simulink model "try1"  (R2013a)
settings: Solver=ode45  StartTime=0.0  StopTime=10.0  RelTol=1e-3
values from neighbouring files (symbols this model uses):
  g = 9.82    [Untitled.m]
  kt = (stall_torque*rm)/max_volt    (= 0.302166666667)    [Untitled.m]
  kv = (stall_torque*rm)/(kt*max_omega)    (= 0.572957795131)    [Untitled.m]
  mp = mtot    (= 2.15528)    [Untitled.m]
  plant = c2d(plant,Ts)    [Untitled.m]
  rm = 7.4    [Untitled.m]
  rp = masscenter    (= 0.156968004157)    [Untitled.m]
undefined symbols (not defined in the file or in its folder): iw, k, kalmanL, kn
libraries: simulink x2
settings Model: Creator=user  LastModifiedBy=user

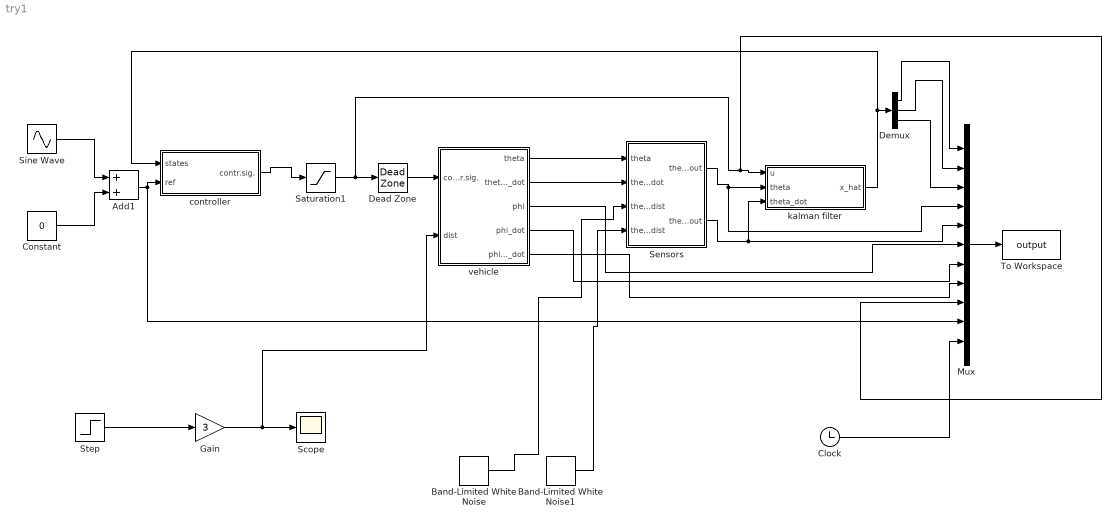
== system try1 ==
  Add1 : Sum
  Band-Limited White Noise : simulink/Sources/Band-Limited White Noise  Cov=[0.1]  Ts=0.1  seed=[23341]
  Band-Limited White Noise1 : simulink/Sources/Band-Limited White Noise  Cov=[0.1]  Ts=0.1  seed=[23341]
  Clock : Clock
  Constant : Constant  Value=0
  Dead Zone : DeadZone  SaturateOnIntegerOverflow=on
  Demux : Demux  Outputs=3
  Gain : Gain  Gain=3
  Mux : Mux  Inputs=11
  Saturation1 : Saturate
  Scope : Scope
  Sensors : Subsystem
  Sine Wave : Sin  SampleTime=0
  Step : Step  SampleTime=0
  To Workspace : ToWorkspace  VariableName=output  SampleTime=-1  SaveFormat=Timeseries
  controller : Subsystem
  kalman filter : Subsystem
  vehicle : Subsystem
  wires:
  Constant/1 -> Add1/2
  Sine Wave/1 -> Add1/1
  Add1/1 -> Mux/10, controller/2(ref)
  vehicle/1(theta) -> Sensors/1(theta)
  vehicle/2(theta_dot) -> Sensors/2(theta_dot)
  Band-Limited White Noise/1 -> Sensors/3(theta_dist)
  Band-Limited White Noise1/1 -> Sensors/4(theta_dot_dist)
  Demux/1 -> Mux/1
  Demux/2 -> Mux/2
  Demux/3 -> Mux/3
  Sensors/1(theta_out) -> Mux/4, kalman filter/2(theta)
  Sensors/2(theta_dot_out) -> kalman filter/3(theta_dot), Mux/5
  controller/1(contr.sig.) -> Saturation1/1
  Mux/1 -> To Workspace/1
  Clock/1 -> Mux/11
  Step/1 -> Gain/1
  Gain/1 -> vehicle/2(dist), Scope/1
  Dead Zone/1 -> vehicle/1(contr.sig.)
  vehicle/3(phi) -> Mux/6
  vehicle/4(phi_dot) -> Mux/7
  vehicle/5(phi_dot_dot) -> Mux/8
  kalman filter/1(x_hat) -> controller/1(states), Demux/1
  Saturation1/1 -> Dead Zone/1, Mux/9, kalman filter/1(u)

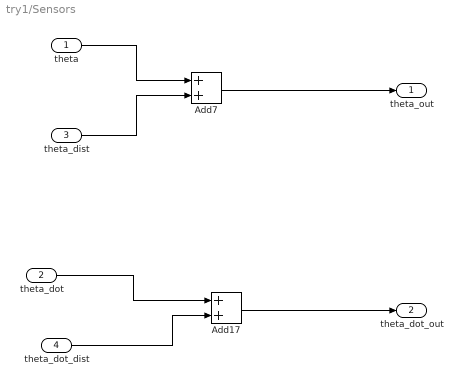
== system try1/Sensors ==
  theta : Inport
  theta_dot : Inport  Port=2
  theta_dist : Inport  Port=3
  theta_dot_dist : Inport  Port=4
  Add17 : Sum
  Add7 : Sum
  theta_out : Outport
  theta_dot_out : Outport  Port=2
  wires:
  theta/1 -> Add7/1
  theta_dist/1 -> Add7/2
  theta_dot/1 -> Add17/1
  theta_dot_dist/1 -> Add17/2
  Add7/1 -> theta_out/1
  Add17/1 -> theta_dot_out/1

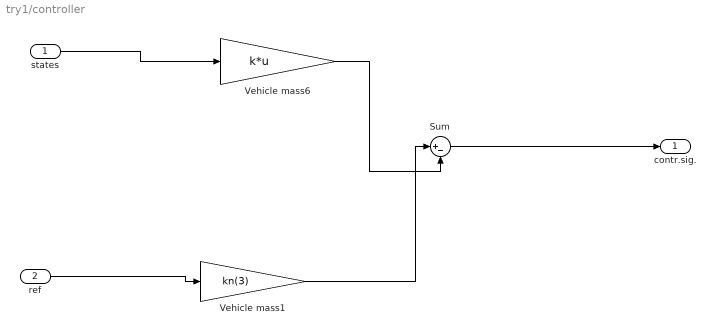
== system try1/controller ==
  states : Inport
  ref : Inport  Port=2
  Sum : Sum  Inputs=|+-
  "Vehicle mass1 " : Gain  Gain=kn(3)
  Vehicle mass6 : Gain  Gain=k*u
  contr.sig. : Outport
  wires:
  ref/1 -> "Vehicle mass1 "/1
  states/1 -> Vehicle mass6/1
  Vehicle mass6/1 -> Sum/2
  "Vehicle mass1 "/1 -> Sum/1
  Sum/1 -> contr.sig./1

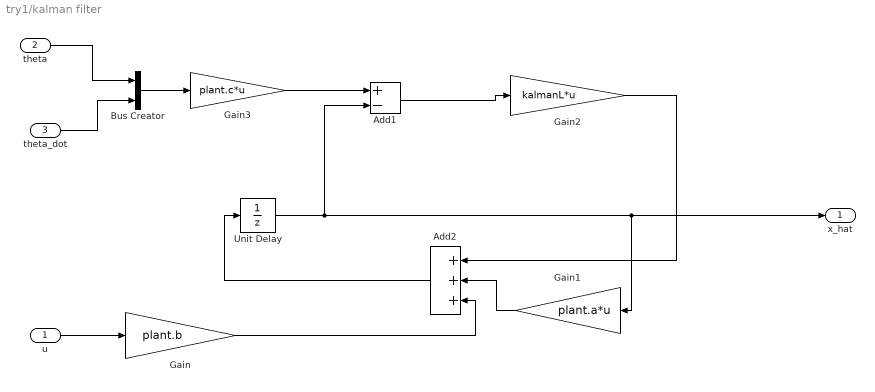
== system try1/kalman filter ==
  u : Inport
  theta : Inport  Port=2
  theta_dot : Inport  Port=3
  Add1 : Sum  Inputs=+-
  Add2 : Sum  Inputs=+++
  Bus Creator : BusCreator  Inputs=2
  Gain : Gain  Gain=plant.b
  Gain1 : Gain  Gain=plant.a*u
  Gain2 : Gain  Gain=kalmanL*u
  Gain3 : Gain  Gain=plant.c*u
  Unit Delay : UnitDelay  SampleTime=-1
  x_hat : Outport
  wires:
  theta/1 -> Bus Creator/1
  theta_dot/1 -> Bus Creator/2
  Bus Creator/1 -> Gain3/1
  Gain3/1 -> Add1/1
  Add1/1 -> Gain2/1
  Gain2/1 -> Add2/1
  Unit Delay/1 -> Add1/2, Gain1/1, x_hat/1
  Add2/1 -> Unit Delay/1
  u/1 -> Gain/1
  Gain/1 -> Add2/3
  Gain1/1 -> Add2/2

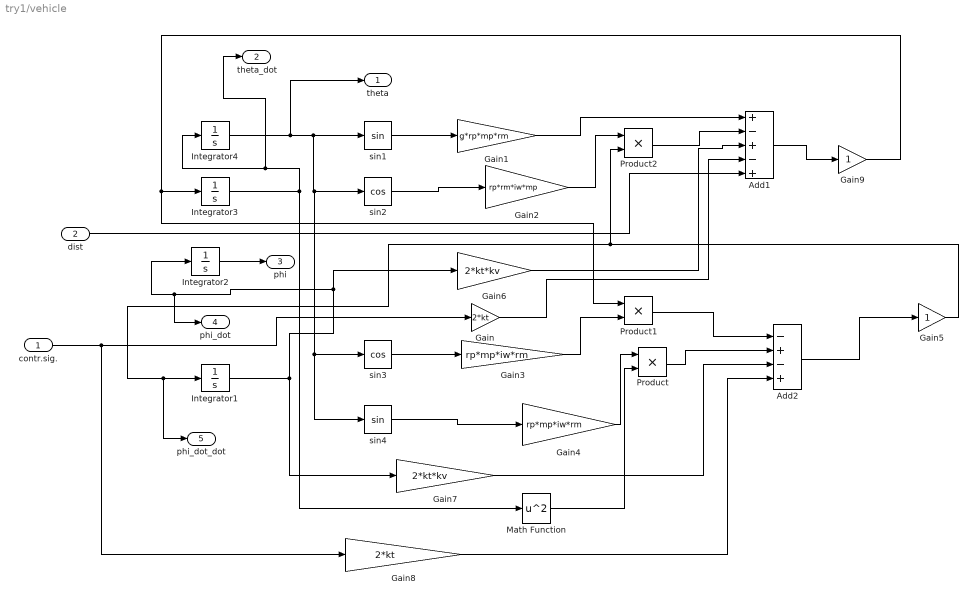
== system try1/vehicle ==
  contr.sig. : Inport
  dist : Inport  Port=2
  Add1 : Sum  Inputs=+-+-+
  Add2 : Sum  Inputs=-+-+
  Gain : Gain  Gain=2*kt
  Gain1 : Gain  Gain=g*rp*mp*rm
  Gain2 : Gain  Gain=rp*rm*iw*mp
  Gain3 : Gain  Gain=rp*mp*iw*rm
  Gain4 : Gain  Gain=rp*mp*iw*rm
  Gain5 : Gain
  Gain6 : Gain  Gain=2*kt*kv
  Gain7 : Gain  Gain=2*kt*kv
  Gain8 : Gain  Gain=2*kt
  Gain9 : Gain
  Integrator{1..4} (4 alike) : Integrator
  Math Function : Math  Operator=square  SaturateOnIntegerOverflow=on
  Product : Product
  Product1 : Product
  Product2 : Product
  sin1 : Trigonometry
  sin2 : Trigonometry  Operator=cos
  sin3 : Trigonometry  Operator=cos
  sin4 : Trigonometry
  theta : Outport
  theta_dot : Outport  Port=2
  phi : Outport  Port=3
  phi_dot : Outport  Port=4
  phi_dot_dot : Outport  Port=5
  wires:
  dist/1 -> Add1/5
  Integrator4/1 -> theta/1, sin4/1, sin3/1, sin2/1, sin1/1
  sin4/1 -> Gain4/1
  sin2/1 -> Gain2/1
  sin1/1 -> Gain1/1
  sin3/1 -> Gain3/1
  Integrator2/1 -> phi/1
  Integrator1/1 -> phi_dot/1, Integrator2/1, Gain6/1, Gain7/1
  Add1/1 -> Gain9/1
  Add2/1 -> Gain5/1
  Gain9/1 -> Integrator3/1, Product1/1
  Gain5/1 -> Product2/2, phi_dot_dot/1, Integrator1/1
  Math Function/1 -> Product/2
  Integrator3/1 -> theta_dot/1, Integrator4/1, Math Function/1
  contr.sig./1 -> Gain8/1, Gain/1
  Gain1/1 -> Add1/1
  Product2/1 -> Add1/2
  Gain2/1 -> Product2/1
  Gain6/1 -> Add1/3
  Gain/1 -> Add1/4
  Gain8/1 -> Add2/4
  Gain7/1 -> Add2/3
  Product1/1 -> Add2/1
  Product/1 -> Add2/2
  Gain4/1 -> Product/1
  Gain3/1 -> Product1/2
